simulink model "TTR_RobustMPC_RTmdl"  (Simulink 8.1)
settings: Solver=ode45  StartTime=0.0  StopTime=10.0  RelTol=1e-3
values from neighbouring files (symbols this model uses):
  TTR_RobustMPC =     [RobustMPC_TTRctrls.mat]    (also in RobustMPC_TTRctrls_INFnorm.mat)
libraries: Robust_MPC_Library x3
settings Model: Creator=Kostas  LastModifiedBy=Kostas
settings DataIOCC: SignalLoggingSaveFormat=Dataset
settings OptimizationCC: ExpressionDepthLimit=128
settings DebuggingCC: FcnCallInpInsideContextMsg=EnableAllAsError
settings GRTTargetCC: CombineOutputUpdateFcns=on  GRTInterface=off

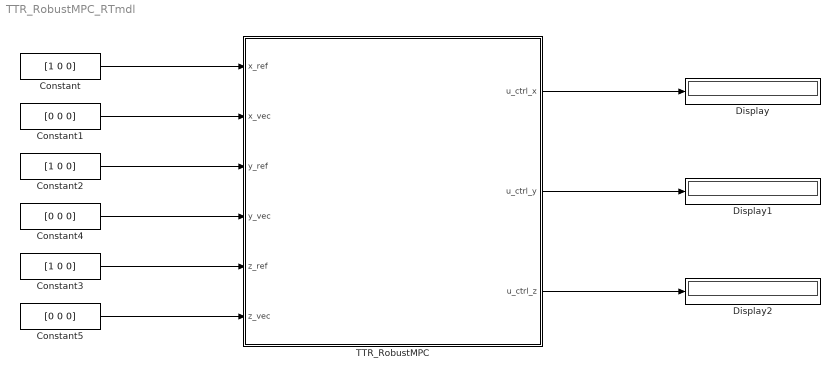
== system TTR_RobustMPC_RTmdl ==
  Constant : Constant  Value=[1 0 0]
  Constant1 : Constant  Value=[0 0 0]
  Constant2 : Constant  Value=[1 0 0]
  Constant3 : Constant  Value=[1 0 0]
  Constant4 : Constant  Value=[0 0 0]
  Constant5 : Constant  Value=[0 0 0]
  Display : Display
  Display1 : Display
  Display2 : Display
  TTR_RobustMPC : Subsystem
  wires:
  Constant/1 -> TTR_RobustMPC/1(x_ref)
  Constant2/1 -> TTR_RobustMPC/3(y_ref)
  Constant3/1 -> TTR_RobustMPC/5(z_ref)
  Constant1/1 -> TTR_RobustMPC/2(x_vec)
  Constant5/1 -> TTR_RobustMPC/6(z_vec)
  TTR_RobustMPC/1(u_ctrl_x) -> Display/1
  TTR_RobustMPC/2(u_ctrl_y) -> Display1/1
  TTR_RobustMPC/3(u_ctrl_z) -> Display2/1
  Constant4/1 -> TTR_RobustMPC/4(y_vec)

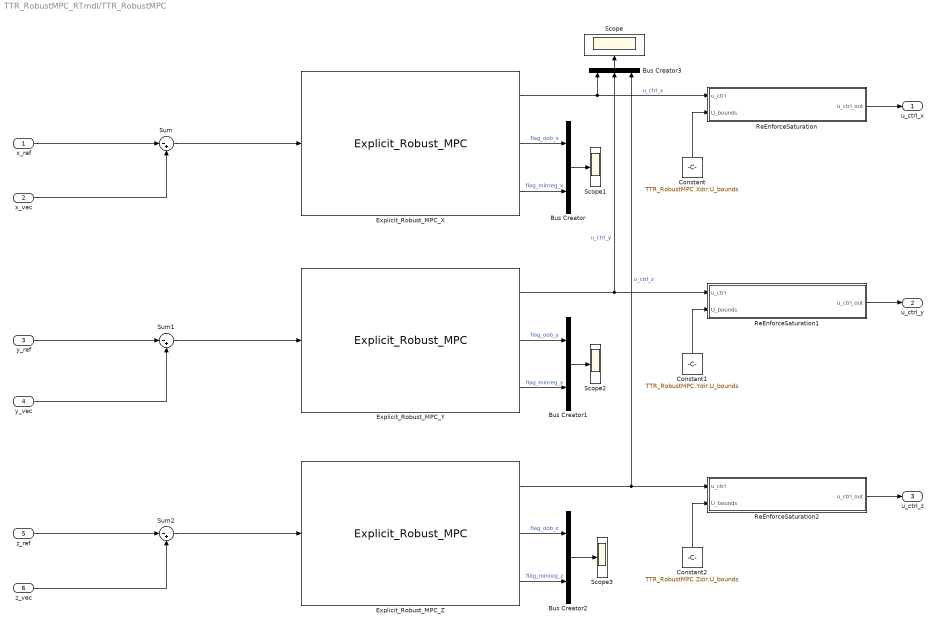
== system TTR_RobustMPC_RTmdl/TTR_RobustMPC ==
  x_ref : Inport
  x_vec : Inport  Port=2
  y_ref : Inport  Port=3
  y_vec : Inport  Port=4
  z_ref : Inport  Port=5
  z_vec : Inport  Port=6
  Bus Creator : BusCreator  Inputs=2
  Bus Creator1 : BusCreator  Inputs=2
  Bus Creator2 : BusCreator  Inputs=2
  Bus Creator3 : BusCreator  Inputs=3
  Constant : Constant  Value=TTR_RobustMPC.Xdir.U_bounds
  Constant1 : Constant  Value=TTR_RobustMPC.Ydir.U_bounds
  Constant2 : Constant  Value=TTR_RobustMPC.Zdir.U_bounds
  Explicit_Robust_MPC_X : Robust_MPC_Library/Explicit_Robust_MPC  H=TTR_RobustMPC.Xdir.H  K=TTR_RobustMPC.Xdir.K  F=TTR_RobustMPC.Xdir.F  G=TTR_RobustMPC.Xdir.G  Nc=TTR_RobustMPC.Xdir.Nc  Nx=TTR_RobustMPC.Xdir.Nx  Hi_init=zeros(100,TTR_RobustMPC.Xdir.Nx)  Ki_init=zeros(100,TTR_RobustMPC.Xdir.Nu)
  Explicit_Robust_MPC_Y : Robust_MPC_Library/Explicit_Robust_MPC  H=TTR_RobustMPC.Ydir.H  K=TTR_RobustMPC.Ydir.K  F=TTR_RobustMPC.Ydir.F  G=TTR_RobustMPC.Ydir.G  Nc=TTR_RobustMPC.Ydir.Nc  Nx=TTR_RobustMPC.Ydir.Nx  Hi_init=zeros(100,TTR_RobustMPC.Ydir.Nx)  Ki_init=zeros(100,TTR_RobustMPC.Ydir.Nu)
  Explicit_Robust_MPC_Z : Robust_MPC_Library/Explicit_Robust_MPC  H=TTR_RobustMPC.Zdir.H  K=TTR_RobustMPC.Zdir.K  F=TTR_RobustMPC.Zdir.F  G=TTR_RobustMPC.Zdir.G  Nc=TTR_RobustMPC.Zdir.Nc  Nx=TTR_RobustMPC.Zdir.Nx  Hi_init=zeros(100,TTR_RobustMPC.Zdir.Nx)  Ki_init=zeros(100,TTR_RobustMPC.Zdir.Nu)
  ReEnforceSaturation : MATLAB Function  TreatAsAtomicUnit=on
  ReEnforceSaturation1 : MATLAB Function  TreatAsAtomicUnit=on
  ReEnforceSaturation2 : MATLAB Function  TreatAsAtomicUnit=on
  Scope{,1..3} (4 alike) : Scope
      Scope settings: SaveName=RobustMPC_uctrl_xyz
      Scope3 settings: SaveName=ScopeData2
  Sum : Sum  Inputs=|-+
  Sum1 : Sum  Inputs=|-+
  Sum2 : Sum  Inputs=|-+
  u_ctrl_x : Outport
  u_ctrl_y : Outport  Port=2
  u_ctrl_z : Outport  Port=3
  wires:
  x_ref/1 -> Sum/1
  x_vec/1 -> Sum/2
  Sum/1 -> Explicit_Robust_MPC_X/1
  Explicit_Robust_MPC_X/1 -> Bus Creator3/1, ReEnforceSaturation/1(u_ctrl)  "u_ctrl_x"
  Sum1/1 -> Explicit_Robust_MPC_Y/1
  y_ref/1 -> Sum1/1
  y_vec/1 -> Sum1/2
  Sum2/1 -> Explicit_Robust_MPC_Z/1
  z_ref/1 -> Sum2/1
  z_vec/1 -> Sum2/2
  ReEnforceSaturation/1(u_ctrl_out) -> u_ctrl_x/1
  Constant/1 -> ReEnforceSaturation/2(U_bounds)
  Explicit_Robust_MPC_Y/1 -> Bus Creator3/2, ReEnforceSaturation1/1(u_ctrl)  "u_ctrl_y"
  Constant1/1 -> ReEnforceSaturation1/2(U_bounds)
  Constant2/1 -> ReEnforceSaturation2/2(U_bounds)
  Explicit_Robust_MPC_Z/1 -> Bus Creator3/3, ReEnforceSaturation2/1(u_ctrl)  "u_ctrl_z"
  ReEnforceSaturation1/1(u_ctrl_out) -> u_ctrl_y/1
  ReEnforceSaturation2/1(u_ctrl_out) -> u_ctrl_z/1
  Explicit_Robust_MPC_X/2 -> Bus Creator/1  "flag_oob_x"
  Explicit_Robust_MPC_X/3 -> Bus Creator/2  "flag_minreg_x"
  Explicit_Robust_MPC_Y/2 -> Bus Creator1/1  "flag_oob_y"
  Explicit_Robust_MPC_Y/3 -> Bus Creator1/2  "flag_minreg_y"
  Explicit_Robust_MPC_Z/2 -> Bus Creator2/1  "flag_oob_z"
  Explicit_Robust_MPC_Z/3 -> Bus Creator2/2  "flag_minreg_z"
  Bus Creator3/1 -> Scope/1
  Bus Creator/1 -> Scope1/1
  Bus Creator1/1 -> Scope2/1
  Bus Creator2/1 -> Scope3/1

== matlab function TTR_RobustMPC/ReEnforceSaturation1 ==
  data: u_ctrl input double; u_ctrl_out output double; U_bounds input double
function u_ctrl_out = ReEnforceSaturations(u_ctrl,U_bounds)
%#codegen

%   this block enforces again the control action saturations. It is not
%   needed and it has been verified that it is not needed. But... you never
%   know. It is always relaxing to be sure that the saturators are enforced
%   whatsoever

u_ctrl_out = u_ctrl;

if length(u_ctrl) ~= (length(U_bounds)/2)
    % that can't be valid! 
    u_ctrl_out = 0; % do something meaningfull hoping that we will save the system...
    flag_inconsistency = 1; % inform the user...
else
    % ok all fine...
    for i = 1:length(u_ctrl)
        u_ctrl_out(i) = max(u_ctrl(i),U_bounds(2*(i-1)+1));
        u_ctrl_out(i) = min(u_ctrl(i),U_bounds(2*(i-1)+2));
    end
end

end

== matlab function TTR_RobustMPC/ReEnforceSaturation ==
  data: u_ctrl input double; u_ctrl_out output double; U_bounds input double
function u_ctrl_out = ReEnforceSaturations(u_ctrl,U_bounds)
%#codegen

%   this block enforces again the control action saturations. It is not
%   needed and it has been verified that it is not needed. But... you never
%   know. It is always relaxing to be sure that the saturators are enforced
%   whatsoever

u_ctrl_out = u_ctrl;

if length(u_ctrl) ~= (length(U_bounds)/2)
    % that can't be valid! 
    u_ctrl_out = 0; % do something meaningfull hoping that we will save the system...
    flag_inconsistency = 1; % inform the user...
else
    % ok all fine...
    for i = 1:length(u_ctrl)
        u_ctrl_out(i) = max(u_ctrl(i),U_bounds(2*(i-1)+1));
        u_ctrl_out(i) = min(u_ctrl(i),U_bounds(2*(i-1)+2));
    end
end

end

== matlab function TTR_RobustMPC/ReEnforceSaturation2 ==
  data: u_ctrl input double; u_ctrl_out output double; U_bounds input double
function u_ctrl_out = ReEnforceSaturations(u_ctrl,U_bounds)
%#codegen

%   this block enforces again the control action saturations. It is not
%   needed and it has been verified that it is not needed. But... you never
%   know. It is always relaxing to be sure that the saturators are enforced
%   whatsoever

u_ctrl_out = u_ctrl;

if length(u_ctrl) ~= (length(U_bounds)/2)
    % that can't be valid! 
    u_ctrl_out = 0; % do something meaningfull hoping that we will save the system...
    flag_inconsistency = 1; % inform the user...
else
    % ok all fine...
    for i = 1:length(u_ctrl)
        u_ctrl_out(i) = max(u_ctrl(i),U_bounds(2*(i-1)+1));
        u_ctrl_out(i) = min(u_ctrl(i),U_bounds(2*(i-1)+2));
    end
end

end
